simulink model "q2"  (R2021a)
settings: Solver=FixedStepAuto  StartTime=0.0  StopTime=10.0  FixedStep=0.001  RelTol=1e-3
undefined symbols (not defined in the file): A, B, C
libraries: cstblocks x3
settings Model: Creator=HASEE  LastModifiedBy=HASEE

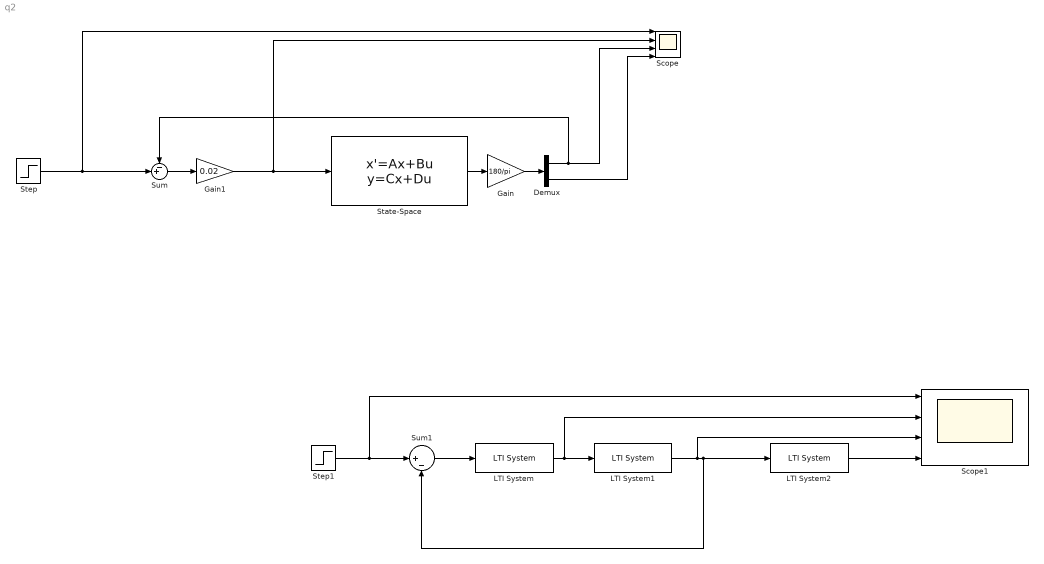
== system q2 ==
  Demux : Demux  Outputs=2
  Gain : Gain  Gain=180/pi
  Gain1 : Gain  Gain=0.02
  LTI System : cstblocks/LTI System  sys=0.02  IC=[]
  LTI System1 : cstblocks/LTI System  sys=Py  IC=[]
  LTI System2 : cstblocks/LTI System  sys=Pt  IC=[]
  Scope : Scope  NumInputPorts=4
  Scope1 : Scope  NumInputPorts=4
  State-Space : StateSpace  A=A  B=B  C=C  D=[0;0]  InitialCondition=0
  Step : Step  Time=0  After=30  SampleTime=0
  Step1 : Step  Time=0  After=30  SampleTime=0
  Sum : Sum  Inputs=-+|
  Sum1 : Sum  Inputs=|+-
  wires:
  Step/1 -> Scope/1, Sum/2
  Sum/1 -> Gain1/1
  Demux/2 -> Scope/4
  State-Space/1 -> Gain/1
  Gain/1 -> Demux/1
  Demux/1 -> Sum/1, Scope/3
  Gain1/1 -> Scope/2, State-Space/1
  LTI System/1 -> Scope1/2, LTI System1/1
  LTI System1/1 -> Scope1/3, LTI System2/1, Sum1/2
  Sum1/1 -> LTI System/1
  LTI System2/1 -> Scope1/4
  Step1/1 -> Scope1/1, Sum1/1
